simulink model "doc_alignment"  (R2014a)
settings: Solver=ode45  StartTime=0.0  StopTime=20  RelTol=1e-3
undefined symbols (not defined in the file or in its folder): commblksprivate, gfprimfd, Info
libraries: dspsigops x2, commblkcod2 x2, commrandsrc2 x1, commsink2 x1
settings Model: CovMetricSettings=d  Creator=The MathWorks Inc.
settings DataIOCC: SignalLoggingSaveFormat=ModelDataLogs  SaveOutput=off  SaveTime=off  SignalLoggingName=logsOut
settings OptimizationCC: BlockReduction=off  BooleanDataType=off  ExpressionDepthLimit=2147483647
settings DebuggingCC: SaveWithParameterizedLinksMsg=none  UnderspecifiedInitializationDetection=Classic  SignalResolutionControl=TryResolveAllWithWarning  SolverPrmCheckMsg=none  MultiTaskDSMMsg=warning  MultiTaskCondExecSysMsg=none  FcnCallInpInsideContextMsg=UseLocalSettings  StateNameClashWarn=warning  StrictBusMsg=None
settings HardwareCC: TargetUnknown=on
settings RTWCC: IncludeERTFirstTime=on
settings GRTTargetCC: TargetFcnLib=iso_c_tmw.mat  CombineOutputUpdateFcns=off  GRTInterface=on

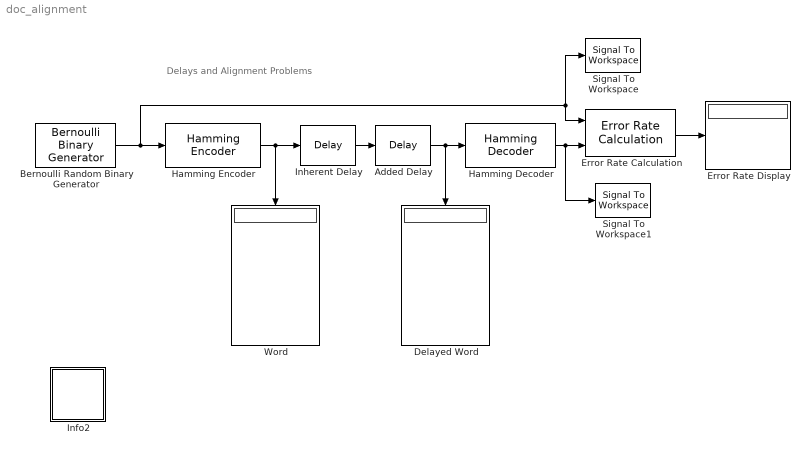
== system doc_alignment ==
  note: Delays and Alignment Problems
  Added Delay : dspsigops/Delay  InputProcessing=Columns as channels (frame based)  dly_unit=Samples  delay=0  ic_detail=off  dif_ic_for_ch=off  dif_ic_for_dly=off  ic=0  reset_popup=None
  Bernoulli Random Binary Generator : commrandsrc2/Bernoulli Binary Generator  P=0.5  seed=89  Ts=1  frameBased=on  sampPerFrame=4  orient=off  outDataType=double
  Delayed Word : Display
  Error Rate Calculation : commsink2/Error Rate Calculation  N=0  st_delay=0  cp_mode=Entire frame  subframe=[]  PMode=Port  WsName=ErrorVec  RsMode2=off  stop=off  numErr=100  maxBits=1e5
  Error Rate Display : Display
  Hamming Decoder : commblkcod2/Hamming Decoder  n=7  k=gfprimfd(3,'min')
  Hamming Encoder : commblkcod2/Hamming Encoder  n=7  k=gfprimfd(3,'min')
  Info2 : Subsystem  AncestorBlock=commblksprivate/Info  mask(Info){}
      settings: OpenFcn=helpview([docroot '/toolbox/comm/comm.map'], 'doc_alignment')
      mask Display: disp('Info')
  Inherent Delay : dspsigops/Delay  InputProcessing=Columns as channels (frame based)  dly_unit=Samples  delay=1  ic_detail=off  dif_ic_for_ch=off  dif_ic_for_dly=off  ic=0  reset_popup=None
  Signal To Workspace : SignalToWorkspace  VariableName=tx
      settings: CopyFcn=dspblkcopystw(gcbh);  Save2DSignal=Inherit from input (this choice will be removed - see release notes)
  Signal To Workspace1 : SignalToWorkspace  VariableName=rx
      settings: CopyFcn=dspblkcopystw(gcbh);  Save2DSignal=Inherit from input (this choice will be removed - see release notes)
  Word : Display
  wires:
  Bernoulli Random Binary Generator/1 -> Hamming Encoder/1, Error Rate Calculation/1, Signal To Workspace/1
  Hamming Decoder/1 -> Error Rate Calculation/2, Signal To Workspace1/1
  Hamming Encoder/1 -> Inherent Delay/1, Word/1
  Inherent Delay/1 -> Added Delay/1
  Error Rate Calculation/1 -> Error Rate Display/1
  Added Delay/1 -> Hamming Decoder/1, Delayed Word/1

== system doc_alignment/Info2 ==
